simulink model "MPC_EKFsimulink"  (R2024a)
settings: Solver=VariableStepAuto  StartTime=0.0  StopTime=10.0  RelTol=1e-3
values from neighbouring files (symbols this model uses):
  p = 20    [EKF.m]    (also in EKFtest.m; MPC_EKF_gpt.m; MPC_with_EKF.m; Q_by_bayesopt.m)
  pvcost = [xf; Q; R; p]    [EKF.m]    (also in EKFtest.m; MPC_EKF_gpt.m; MPC_with_EKF.m; Q_by_bayesopt.m = [xf; best_Q; R; p])
  pvstate = ParamTable.Value    [EKF.m]    (also in EKFtest.m; MPC_EKF_gpt.m; MPC_with_EKF.m; Q_by_bayesopt.m)
  u0 = zeros(nmv,1)    [EKF.m]    (also in EKFtest.m; MPC_EKF_gpt.m; MPC_with_EKF.m; Q_by_bayesopt.m)
  x0 = [0.2618; 0; 0; 0]    [EKF.m]    (also in EKFtest.m = [0.0873; 0; 0; 0]; MPC_EKF_gpt.m = [0.0873; 0; 0; 0]; MPC_with_EKF.m = [0.0873; 0; 0; 0]; Q_by_bayesopt.m = [0.0873; 0; 0; 0])
libraries: mpclib x1
settings Model: Creator=soshi  LastModifiedBy=soshi

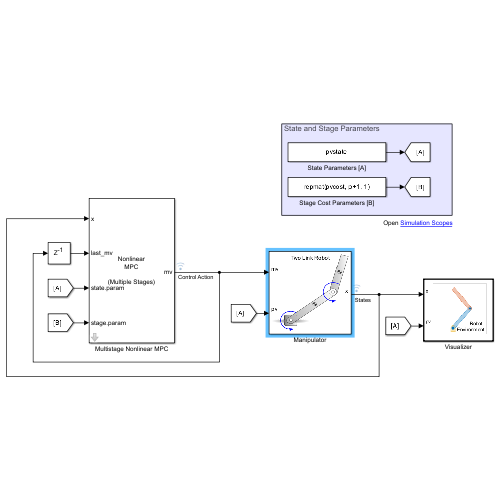
[thumbnail: Simulink's stored preview of the top-level diagram]
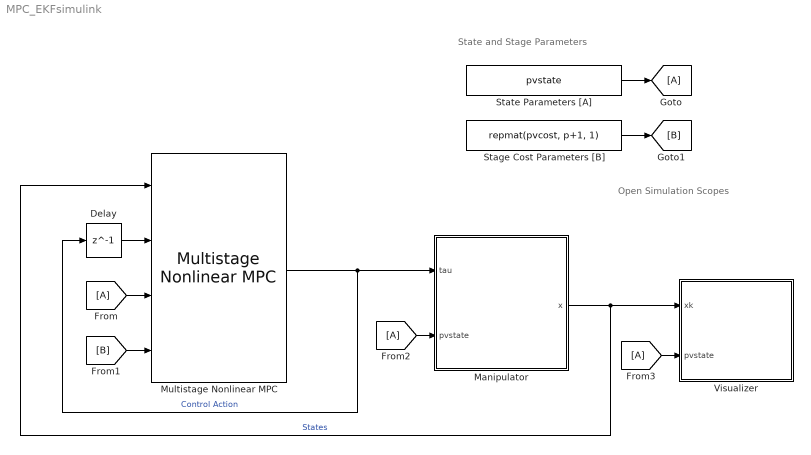
== system MPC_EKFsimulink ==
  note: State and Stage Parameters
  note: Open Simulation Scopes
  Delay : Delay  DelayLength=1  InitialCondition=u0
  From : From
  From2 : From
  From3 : From
  Goto : Goto
  Manipulator : Subsystem
  Multistage Nonlinear MPC : mpclib/Multistage Nonlinear MPC  nlmpcobj=msobj  UseObjectTs=on  TsControl=-1  UseMEX=on  mexname=nlmpcControllerMEX  md_enabled=off  stateparam_enabled=on  stageparam_enabled=on  cost_enabled=off  mvseq_enabled=off  stateseq_enabled=off  slack_enabled=off  status_enabled=off  mv_min=off  mv_max=off  mvrate_min=off  mvrate_max=off  state_min=off  state_max=off  terminal_state=off  nlp_initialize=off
  Stage Cost Parameters [B] : Constant  Value=repmat(pvcost, p+1, 1)  VectorParams1D=off
  State Parameters [A] : Constant  Value=pvstate  VectorParams1D=off
  Visualizer : MATLAB Function  TreatAsAtomicUnit=on
  wires:
  Stage Cost Parameters [B]/1 -> [B]
  State Parameters [A]/1 -> Goto/1
  From3/1 -> Visualizer/2(pvstate)
  [B] -> Multistage Nonlinear MPC/4
  From/1 -> Multistage Nonlinear MPC/3
  From2/1 -> Manipulator/2(pvstate)
  Manipulator/1(x) -> Visualizer/1(xk), Multistage Nonlinear MPC/1  "States"
  Delay/1 -> Multistage Nonlinear MPC/2
  Multistage Nonlinear MPC/1 -> Delay/1, Manipulator/1(tau)  "Control Action"

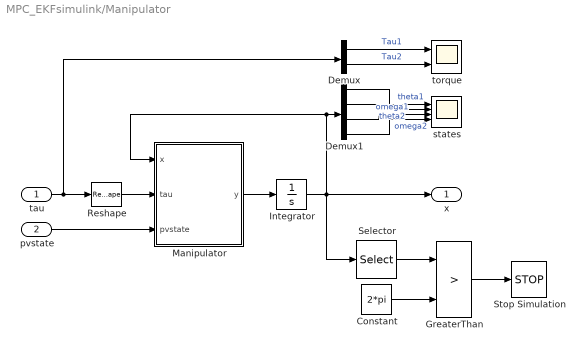
== system MPC_EKFsimulink/Manipulator ==
  tau : Inport
  pvstate : Inport  Port=2
  Constant : Constant  Value=2*pi
  Demux : Demux  Outputs=2
  Demux1 : Demux
  GreaterThan : RelationalOperator  Operator=>  OutDataTypeStr=boolean  RndMeth=Simplest  InputSameDT=off
  Integrator : Integrator  InitialCondition=x0
  Manipulator : MATLAB Function  TreatAsAtomicUnit=on
  Reshape : Reshape  OutputDimensionality=Customize  OutputDimensions=[2,1]
  Selector : Selector  InputPortWidth=4  IndexOptions=Index vector (dialog)  Indices=1  OutputSizes=1
  Stop Simulation : Stop
  states : Scope  NumInputPorts=4
  torque : Scope  NumInputPorts=2
  x : Outport
  wires:
  Manipulator/1(y) -> Integrator/1
  tau/1 -> Demux/1, Reshape/1
  Reshape/1 -> Manipulator/2(tau)
  Integrator/1 -> Selector/1, x/1, Manipulator/1(x), Demux1/1
  GreaterThan/1 -> Stop Simulation/1
  Constant/1 -> GreaterThan/2
  Selector/1 -> GreaterThan/1
  pvstate/1 -> Manipulator/3(pvstate)
  Demux1/4 -> states/4  "omega2"
  Demux/1 -> torque/1  "Tau1"
  Demux1/1 -> states/1  "theta1"
  Demux1/3 -> states/3  "omega1"
  Demux1/2 -> states/2  "theta2"
  Demux/2 -> torque/2  "Tau2"

== matlab function MPC_EKFsimulink/Manipulator/Manipulator ==
  data: x input; tau input; y output; pvstate input
function y = fcn(x, tau, pvstate)
y = twolinkStateFcn(x, tau, pvstate);

== matlab function MPC_EKFsimulink/Visualizer ==
  data: xk input; xf parameter; pvstate input
function fcn(xk, xf, pvstate)
% This function launches the Robot Environment that animates a two-link
% robot during Simulink simulation. It takes the current state (xk),
% desired state (xf), and physical parameters for the robot (pvstate) as
% inputs.

% Declare PlotTwoLinkRobot.simulinkPlot function as an extrinsic function.
coder.extrinsic('helperRobotEnvironment.simulinkPlot');

% Update Robot Environment
helperRobotEnvironment.simulinkPlot(xk, xf, pvstate)
